simulink model "final_part3"  (R2023a)
settings: Solver=ode1  StartTime=0.0  StopTime=999  FixedStep=0.001  RelTol=1e-3  EnableMultiTasking=on
values from neighbouring files (symbols this model uses):
  a = 81.44    [DetermineTorqConstants.m]    (also in part4.m = 69.9384142006)
  A = [ 0 1 0 0 ... (first row only)    [part4.m]    (also in untitled2.m = [1;0])
  B = [ 0; -0.87; 0; 163]    [part4.m]
  C = [1 0 0 0 ; 0 0 1 0]    [part4.m]
  K = place (A,B, p)    [part4.m]
  K_unstable = place (A_d,B, p_unstable)    [part4.m]
undefined symbols (not defined in the file or in its folder): L
libraries: c6xlib x6, fricblocks x3
Description:
  | Real-Time Van der Pol Simulation
  | 
  | This demonstration shows a real-time version of the Simulink(R) Van der Pol
  | simulation demo. This model does not need any external signals, so it does
  | not need any data acquisition hardware or driver. This makes the model ideal
  | for first experiments with Real-Time Windows Target(TM), without need to
  | worry about proper I/O hardware configuration.
  | 
  | How to run this demo:
  | 
  |   1. Build the model using Tools -> Real-Time Workshop -> Build Model.
  |   2. Connect to the real-time code using Simulation -> Connect to target.
  |   3. Start the real-time execution using Simulation -> Start real-time code.
settings Model: SimulationMode=external  ExtModeTrigDuration=50000  Creator=Houska  LastModifiedBy=rawnies2
settings SolverCC: AlgebraicLoopSolver=TrustRegion
settings DataIOCC: LimitDataPoints=on  SaveFormat=Array  SignalLoggingSaveFormat=ModelDataLogs  ReturnWorkspaceOutputs=off  SignalLoggingName=logsOut
settings OptimizationCC: ExpressionDepthLimit=2147483647  InitFltsAndDblsToZero=on  EfficientMapNaN2IntZero=off
settings DebuggingCC: UnderspecifiedInitializationDetection=Classic  MergeDetectMultiDrivingBlocksExec=none  SignalResolutionControl=TryResolveAllWithWarning  FcnCallInpInsideContextMsg=warning  UnconnectedInputMsg=warning  UnconnectedOutputMsg=warning  UnconnectedLineMsg=warning  StateNameClashWarn=warning  SFUnexpectedBacktrackingDiag=warning  SFNoUnconditionalDefaultTransitionDiag=warning  SFExecutionAtInitializationDiag=none  ArithmeticOperatorsInVariantConditions=warning
settings HardwareCC: ProdBitPerLong=64  ProdHWDeviceType=Intel->x86-64 (Linux 64)  TargetIntDivRoundTo=Zero  TargetEndianess=LittleEndian  TargetHWDeviceType=Intel->x86/Pentium
settings ModelReferenceCC: EnableRefExpFcnMdlSchedulingChecks=on  PropagateSignalLabelsOutOfModel=off
settings SFSimCC: SimUseLocalCustomCode=off  CustomCodeUndefinedFunction=UseInterfaceOnly
settings RTWCC: Description=Simulink Desktop Real-Time  SystemTargetFile=sldrt.tlc  TemplateMakefile=sldrt.tmf  RTWUseLocalCustomCode=off  RTWCompilerOptimization=on
settings CodeAppCC: MaxIdLength=95  StateflowObjectComments=on
settings SimulinkDesktopRealTimeCC: TargetLibSuffix=_sldrt.a  TargetPreCompLibLocation=C:\MATLABR2023a\toolbox\sldrt\lib\win64  TargetLangStandard=C89/C90 (ANSI)  SupportVariableSizeSignals=off
settings ConfigComp: CovMetricSettings=dw  CovSaveCumulativeToWorkspaceVar=on  CovSaveSingleToWorkspaceVar=on  CovExternalEMLEnable=off  CovSFcnEnable=off

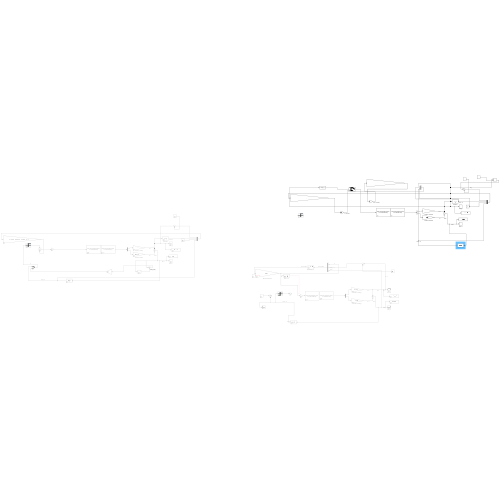
[thumbnail: Simulink's stored preview of the top-level diagram]
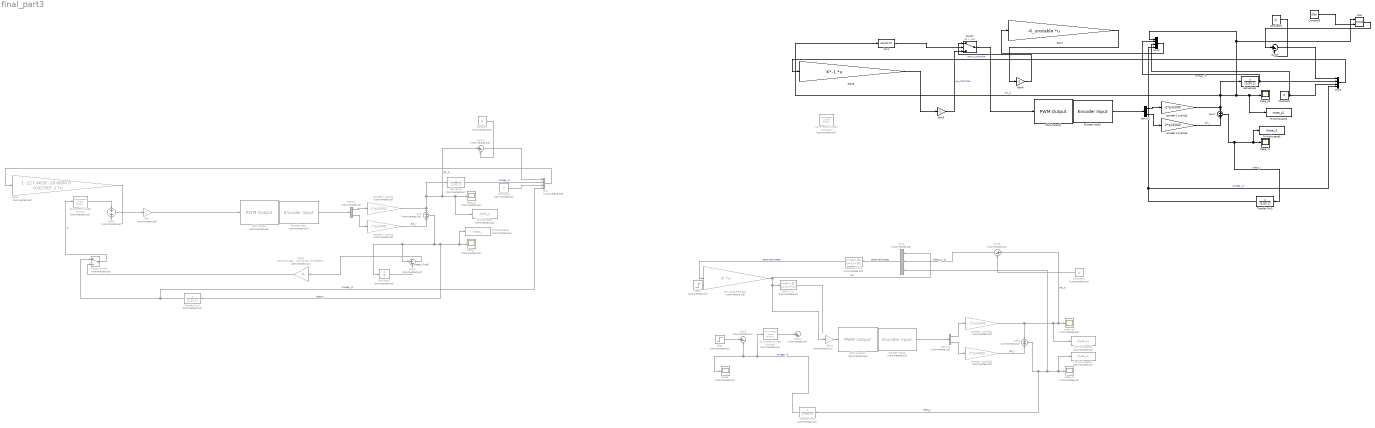
== system final_part3 ==
  note: theta_r(t-dt)
  Asymmetric Linear Friction : fricblocks/Asymmetric  Linear Friction  Commented=on  intercept1=0.6043  intercept2=-0.6143  slope1=0.01219  slope2=0.01291
  Asymmetric Linear Friction1 : fricblocks/Asymmetric  Linear Friction  Commented=on  intercept1=0.6043  intercept2=-0.6143  slope1=0.01219  slope2=0.01291
  Asymmetric Linear Friction2 : fricblocks/Asymmetric  Linear Friction  Commented=on  intercept1=0.6043  intercept2=-0.6143  slope1=0.01219  slope2=0.01291
  Constant : Constant  Commented=on  Value=pi
  Constant1 : Constant  Commented=on  Value=0
  Constant2 : Constant  Commented=on  Value=pi
  Constant3 : Constant  Value=pi
  Constant4 : Constant  Value=0
  Constant5 : Constant  Value=2*pi
  Demux : Demux  Commented=on  Outputs=2
  Demux1 : Demux  Commented=on  Outputs=2
  Demux2 : Demux  Outputs=2
  Encoder Input : c6xlib/Encoder Input  Commented=on  baseAddr=findParallelAddress  channels=[0 1]  sampleTime=str2num(get_param(bdroot, 'FixedStep'))
  Encoder Input1 : c6xlib/Encoder Input  Commented=on  baseAddr=findParallelAddress  channels=[0 1]  sampleTime=str2num(get_param(bdroot, 'FixedStep'))
  Encoder Input2 : c6xlib/Encoder Input  baseAddr=findParallelAddress  channels=[0 1]  sampleTime=str2num(get_param(bdroot, 'FixedStep'))
  Fcn1 : Fcn  Expr=cos(u(1))
  Gain : Gain  Commented=on  Gain=-1
  Gain1 : Gain  Commented=on  Gain="[ -227.4626  -18.6600   0   -0.0278]*-1"  Multiplication=Matrix(K*u) (u vector)
  Gain2 : Gain  Commented=on  Gain=1/str2num(get_param(bdroot, 'FixedStep'))
  Gain3 : Gain  Gain=-1
  Gain4 : Gain  Commented=on  Gain=-1
  Gain5 : Gain  Gain=K*-1  Multiplication=Matrix(K*u) (u vector)
  Gain7 : Gain  Gain=-K_unstable  Multiplication=Matrix(K*u) (u vector)
  Gain8 : Gain  Gain=-1
  Manual Switch : ManualSwitch  Commented=on
  Mod : Math  Operator=mod
  Mux : Mux  Commented=on
  Mux1 : Mux  Commented=on  Inputs=3
  Mux2 : Mux
  Mux3 : Mux
  PWM Output : c6xlib/PWM Output  Commented=on  baseAddr=findParallelAddress  channels=0  initialOutputs=0  finalOutputs=0  sampleTime=str2num(get_param(bdroot, 'FixedStep'))
  PWM Output1 : c6xlib/PWM Output  Commented=on  baseAddr=findParallelAddress  channels=0  initialOutputs=0  finalOutputs=0  sampleTime=str2num(get_param(bdroot, 'FixedStep'))
  PWM Output2 : c6xlib/PWM Output  baseAddr=findParallelAddress  channels=0  initialOutputs=0  finalOutputs=0  sampleTime=str2num(get_param(bdroot, 'FixedStep'))
  RWP (4.1) : StateSpace  Commented=on  A="[ 0 1  ; a 0 ];"  B=[ 0; -0.87];  C=[ 0 0;0 0]  D=[ 0 ;0]  InitialCondition=0
  Scope : Scope  Commented=on
  Step : Step  Commented=on  Time=0  After=5  SampleTime=0
  Step1 : Step  Commented=on  Time=0  After=5  SampleTime=0
  Sum : Sum  Commented=on
  Sum{1,3,5,8} (4 alike) : Sum  Commented=on  Inputs=|+-
  Sum2 : Sum  Commented=on
  Sum4 : Sum  Commented=on
  Sum6 : Sum  Commented=on  Inputs=|++
  Sum7 : Sum
  Sum9 : Sum  Inputs=|+-
  Switch : Switch  Criteria=u2 > Threshold  Threshold=-0.4  SaturateOnIntegerOverflow=off  InputSameDT=off
  To Workspace : ToWorkspace  Commented=on  VariableName=theta_p  SaveFormat=Structure With Time  SampleTime=-1
  To Workspace1 : ToWorkspace  Commented=on  VariableName=theta_r  SaveFormat=Structure With Time  SampleTime=-1
  To Workspace2 : ToWorkspace  Commented=on  VariableName=theta_p1  SaveFormat=Structure With Time  SampleTime=-1
  To Workspace3 : ToWorkspace  Commented=on  VariableName=theta_r1  SaveFormat=Structure With Time  SampleTime=-1
  To Workspace4 : ToWorkspace  VariableName=theta_p2  SaveFormat=Structure With Time  SampleTime=-1
  To Workspace5 : ToWorkspace  VariableName=theta_r2  SaveFormat=Structure With Time  SampleTime=-1
  Transfer Fcn1 : TransferFcn  Commented=on  Numerator=[1 0]  Denominator=[1/50 1]
  Transfer Fcn2 : TransferFcn  Commented=on  Numerator=[1 0]  Denominator=[1/50 1]
  Transfer Fcn3 : TransferFcn  Numerator=[1 0]  Denominator=[1/50 1]
  Unit Delay : UnitDelay  Commented=on  SampleTime=-1  HasFrameUpgradeWarning=on
  derivative : TransferFcn  Commented=on  Numerator=[1 0]  Denominator=[1/50 1]
  derivative1 : TransferFcn  Numerator=[1 0]  Denominator=[1/50 1]
  encoder 1 scaling : Gain  Commented=on  Gain=-2*pi/5000
  encoder 1 scaling1 : Gain  Commented=on  Gain=-2*pi/5000
  encoder 1 scaling2 : Gain  Gain=-2*pi/5000
  encoder 2 scaling : Gain  Commented=on  Gain=2*pi/4000
  encoder 2 scaling1 : Gain  Commented=on  Gain=2*pi/4000
  encoder 2 scaling2 : Gain  Gain=2*pi/4000
  observer (5.1)1 : StateSpace  Commented=on  A=A-L*C  B=[B L]  C=eye(4)  D=zeros(4, 3)  InitialCondition=0  ParameterTunability=Unconstrained
  still using RWP gain : Gain  Commented=on  Gain=-K  Multiplication=Matrix(K*u) (u vector)
  theta_p : Scope  Commented=on
  theta_p1 : Scope  Commented=on
  theta_p2 : Scope
  theta_r : Scope  Commented=on
  theta_r1 : Scope  Commented=on
  theta_r2 : Scope
  wires:
  Demux/1 -> encoder 1 scaling/1
  Demux/2 -> encoder 2 scaling/1
  encoder 1 scaling/1 -> To Workspace/1, theta_p/1, Sum1/1, derivative/1, Sum/1  "phi_p"
  encoder 2 scaling/1 -> Sum/2  "phi_r"
  Encoder Input/1 -> Demux/1
  Sum/1 -> Sum3/1, Unit Delay/1, Transfer Fcn1/1, To Workspace1/1, theta_r/1  "theta_r"
  Gain/1 -> PWM Output/1
  Unit Delay/1 -> Sum3/2
  Sum3/1 -> Gain2/1
  Manual Switch/1 -> Asymmetric Linear Friction/1  "w"
  Gain2/1 -> Manual Switch/2
  Transfer Fcn1/1 -> Mux/4, Manual Switch/1  "omega _R"
  Asymmetric Linear Friction/1 -> Sum2/1
  Constant/1 -> Sum1/2
  Sum1/1 -> Mux/1
  Constant1/1 -> Mux/3
  Mux/1 -> Gain1/1
  Gain1/1 -> Sum2/2
  Sum2/1 -> Gain/1
  derivative/1 -> Mux/2  "omega _R"
  Step1/1 -> ?
  RWP (4.1)/1 -> ?
  Demux1/1 -> encoder 1 scaling1/1
  Encoder Input1/1 -> Demux1/1
  still using RWP gain/1 -> Mux1/1, RWP (4.1)/1, Gain4/1  "-Ku"
  Asymmetric Linear Friction1/1 -> Sum6/1
  Step/1 -> Sum5/1
  Transfer Fcn2/1 -> Asymmetric Linear Friction1/1, Scope/1, Sum5/2  "omega _R"
  Gain4/1 -> PWM Output1/1
  Constant2/1 -> Sum8/2
  encoder 1 scaling1/1 -> Sum4/1, To Workspace2/1, Sum8/1, theta_p1/1  "phi_p"
  Demux1/2 -> encoder 2 scaling1/1
  encoder 2 scaling1/1 -> Sum4/2  "phi_r"
  Sum4/1 -> Mux1/3, To Workspace3/1, theta_r1/1, Transfer Fcn2/1  "theta_r"
  Mux1/1 -> observer (5.1)1/1  "observed states"
  observer (5.1)1/1 -> still using RWP gain/1  "observed states"
  Sum8/1 -> Mux1/2  "theta_p - pi"
  Transfer Fcn3/1 -> Mux2/4, Mux3/4  "omega _R"
  Demux2/1 -> encoder 1 scaling2/1
  Demux2/2 -> encoder 2 scaling2/1
  encoder 1 scaling2/1 -> To Workspace4/1, theta_p2/1, Mod/1, Mux3/1, Fcn1/1, derivative1/1, Sum7/1  "phi_p"
  encoder 2 scaling2/1 -> Sum7/2  "phi_r"
  Switch/1 -> PWM Output2/1
  Fcn1/1 -> Switch/2
  Mux3/1 -> Gain7/1
  Encoder Input2/1 -> Demux2/1
  Constant3/1 -> Sum9/2
  Sum7/1 -> Transfer Fcn3/1, To Workspace5/1, theta_r2/1  "theta_r"
  Constant4/1 -> Mux3/3, Mux2/3
  Gain7/1 -> Gain8/1
  Sum9/1 -> Mux2/1
  Mux2/1 -> Gain5/1
  derivative1/1 -> Mux3/2, Mux2/2  "omega _R"
  Gain3/1 -> Switch/3  "up_controller"
  Gain8/1 -> Switch/1  "down_controller"
  Constant5/1 -> Mod/2
  Gain5/1 -> Gain3/1
  Mod/1 -> Sum9/1
